simulink model "sim_autotrans"  (R2018b)
settings: Solver=ode5  StartTime=0.0  StopTime=30  RelTol=1e-3  AbsTol=1e-6
PostLoadFcn:
  | removeModelListener(bdroot(gcs))
InitFcn:
  | [listenerNodes] = setupModelListener(gcs);
StopFcn:
  | runModelCoverage(gcs,listenerNodes,dataObj,ChartObj,stateFlowCov,groupCharts,1)
model workspace (MAT data in the model file):
  CONVERTER_DATA = [0  137.465208994  2.232; 0.1  137.065019157  2.075; 0.2  135.864449646  1.975; 0.3  135.664354728  1.846; 0.4  137.565256453  1.72; 0.5  140.366585312  1.564; 0.6  145.268910814  1.409; 0.7  152.872517717  1.254; 0.8  162.9773111  1.096; 0.81  164.27792807  1.08; 0.82  166.178829795  1.061; 0.83  167.979684062  1.043; 0.84  170.080680706  1.028; 0.85  172.781962105  1.012; 0.86  175.383196045  1.002; 0.87  179.585189333  1.002; 0.88  183.587087703  1.001; 0.89  189.890077635  0.998; 0.9  197.693779455  0.999; 0.92  215.902417037  1.001; 0.94  244.515990379  1.002]
  DOWN_TABLE = [0  5  20  35; 0  5  20  35; 0  5  25  40; 0  5  30  50; 0  30  50  80; 0  30  50  80]
  DOWN_TH_BP = [0; 5; 40; 50; 90; 100]
  EMAP = [-40  -44  -49  -53  -57  -61  -65  -70  -74  -78  -82; 215  117  85  66  44  29  10  -2  -13  -22  -32; 245  208  178  148  122  104  85  66  48  33  18; 264  260  241  219  193  167  152  133  119  96  85; 264  279  282  275  260  238  223  208  189  171  152; 267  290  293  297  290  275  260  256  234  212  193; 267  297  305  305  305  301  293  282  267  249  226; 267  301  308  312  319  323  319  316  297  279  253; 267  301  312  319  327  327  327  327  312  293  267; 267  301  312  319  327  334  334  334  319  305  275]
  Iei = 0.0219914882836
  NE_VEC = [800 1200 1600 2000 2400 2800 3200 3600 4000 4400 4800]
  TH_VEC = [0; 20; 30; 40; 50; 60; 70; 80; 90; 100]
  TWAIT = 2
  UP_TABLE = [10  30  50  1000000; 10  30  50  1000000; 15  30  50  1000000; 23  41  60  1000000; 40  70  100  1000000; 40  70  100  1000000]
  UP_TH_BP = [0; 25; 35; 50; 90; 100]
  VEHICLE_DATA = [3.23; 40; 0.02; 1; 12.0941478573; 0]
undefined symbols (not defined in the file): sigbuilder_block
Description:
  | Modeling an Automatic Transmission Controller
  | 
  | In this example, Simulink(R) is used to model an automotive drivetrain. Stateflow(R)
  | enhances the Simulink model with its representation of the transmission
  | control logic. Simulink provides a powerful environment for the modeling and
  | simulation of dynamic systems and processes. In many systems, though,
  | supervisory functions like changing modes or invoking new gain schedules must
  | respond to events that may occur and conditions that develop over time. As a
  | result, the environment requires a language capable of managing these multiple
  | modes and developing conditions. In the following example, Stateflow
  | demonstrates its strength in this capacity by performing the function of gear
  | selection in an automatic transmission. This function is combined with the
  | drivetrain dynamics in a natural and intuitive manner by incorporating a
  | Stateflow block in the Simulink block diagram.
settings Model: DataTypeOverride=Double  MinMaxOverflowLogging=ForceOff  FPTRunName=Active  PauseTimes=15  ExtModeTrigMode=oneshot  ExtModeArmWhenConnect=off  ExtModeAutoUpdateStatusClock=off  Creator=The MathWorks, Inc.  LastModifiedBy=nacnm6
settings SolverCC: AutoScaleAbsTol=off
settings DataIOCC: SaveFormat=StructureWithTime  SaveOutput=off  SaveTime=off  SignalLoggingName=Harness_Signal_Log
settings OptimizationCC: BlockReduction=off  ExpressionDepthLimit=2147483647  InitFltsAndDblsToZero=on  LifeSpan=inf
settings DebuggingCC: SignalInfNanChecking=error  ReadBeforeWriteMsg=DisableAll  WriteAfterWriteMsg=DisableAll  WriteAfterReadMsg=DisableAll  SaveWithParameterizedLinksMsg=none  CheckExecutionContextPreStartOutputMsg=on  CheckExecutionContextRuntimeOutputMsg=on  MultiTaskCondExecSysMsg=none  SigSpecEnsureSampleTimeMsg=none  IntegerOverflowMsg=none  FcnCallInpInsideContextMsg=warning  SignalLabelMismatchMsg=error  UnconnectedInputMsg=error  UnconnectedOutputMsg=error  UnconnectedLineMsg=error  UniqueDataStoreMsg=error  BusObjectLabelMismatch=error  RootOutportRequireBusObject=error  AllowSymbolicDim=off  StateNameClashWarn=warning  StrictBusMsg=ErrorOnBusTreatedAsVector  NonBusSignalsTreatedAsBus=error  SFUnexpectedBacktrackingDiag=warning  SFNoUnconditionalDefaultTransitionDiag=warning  SFExecutionAtInitializationDiag=none  IntegerSaturationMsg=none
settings HardwareCC: ProdBitPerPointer=32  ProdBitPerSizeT=32  ProdBitPerPtrDiffT=32  ProdLargestAtomicFloat=None  ProdIntDivRoundTo=Floor  ProdEndianess=Unspecified  ProdWordSize=32  ProdHWDeviceType=32-bit Generic
settings ModelReferenceCC: PropagateSignalLabelsOutOfModel=off
settings SFSimCC: SFSimEcho=off  SimUseLocalCustomCode=off  SimParseCustomCode=off
settings RTWCC: RTWUseLocalCustomCode=off
settings CodeAppCC: StateflowObjectComments=on
settings GRTTargetCC: TargetFcnLib=ansi_tfl_tmw.mat  TargetLangStandard=C89/C90 (ANSI)  GeneratePreprocessorConditionals=Disable all  CombineOutputUpdateFcns=off  GRTInterface=on
settings ConfigComp: CovMetricSettings=dcmtr  CovHTMLOptions=-aTS=1 -bRG=1 -bTC=1 -hTR=0 -nFC=0 -scm=1 -bcm=1 -xEv=0  CovSaveCumulativeToWorkspaceVar=on  CovSaveSingleToWorkspaceVar=on  CovExternalEMLEnable=off

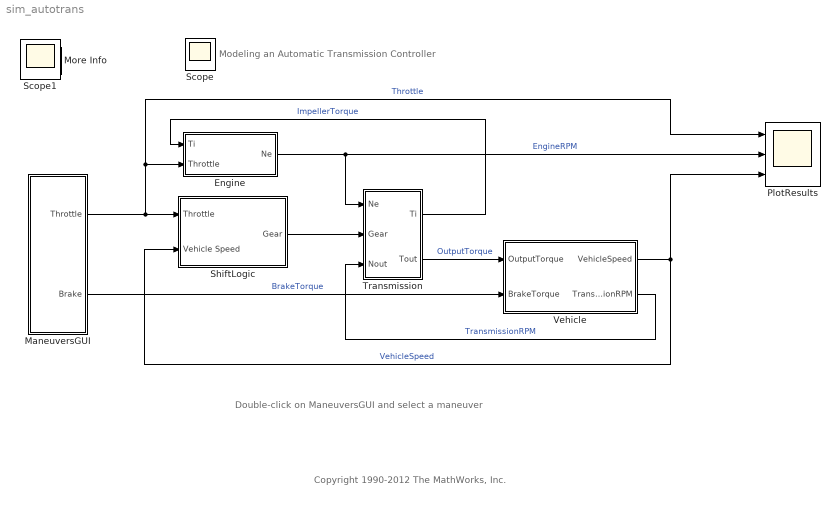
== system sim_autotrans ==
  note: Double-click on ManeuversGUI and select a maneuver
  note: Modeling an Automatic Transmission Controller
  note: Copyright 1990-2012 The MathWorks, Inc.
  Engine : Subsystem
  ManeuversGUI : Subsystem  Tag=STV Subsys  LoadFcn=sigbuilder_block('load');  StartFcn=sigbuilder_block('start');  StopFcn=sigbuilder_block('stop');  ClipboardFcn=sigbuilder_block('clipboard');  mask(Sigbuilder block){tuvar=[0:10]}
      mask help: Sigbuilder GUI
      mask init:
      | tuvar = sigbuilder_block('maskInit');
      settings: CopyFcn=sigbuilder_block('copy');  DeleteFcn=sigbuilder_block('delete');  ModelCloseFcn=sigbuilder_block('modelClose');  PreSaveFcn=sigbuilder_block('preSave');  PauseFcn=sigbuilder_block('pause')  ContinueFcn=sigbuilder_block('continue')  NameChangeFcn=sigbuilder_block('namechange');  OpenFcn=sigbuilder_block('open',[80.8 328 413.6 257.6 ]);  CloseFcn=sigbuilder_block('close');
      mask Display: plot(0, 0, 100, 100,[2, 2, 32, 32, 2], [68, 8, 8, 68, 68],[32, 2], [38, 38], [32, 19, 2],[53, 60, 44], [32, 17, 17, 2],[16, 16, 31, 31]);txt = getActiveGroup(gcbh);text(2, 100, txt,'verticalAlignment', 'top');
  More Info : Subsystem
      settings: OpenFcn=showdemo(bdroot(gcb))
      mask Display: disp('?')
  PlotResults : Scope  NumInputPorts=3
  ShiftLogic : Subsystem  TreatAsAtomicUnit=on  SystemSampleTime=0.04
  Transmission : Subsystem
  Vehicle : Subsystem  mask(vehicle model){Rfd=VEHICLE_DATA(1), rload0=VEHICLE_DATA(2), rload2=VEHICLE_DATA(3), Rw=VEHICLE_DATA(4), Iv=VEHICLE_DATA(5), N20=VEHICLE_DATA(6)/VEHICLE_DATA(4)*VEHICLE_DATA(1)}
      mask prompts: Rfd "final drive ratio"; rload0 "drag friction at wheels"; rload2 "aerodynamic drag"; Rw "wheel radius"; Iv "vehicle inertia"; N20 "initial transmission output speed"
      mask help: vehicle dynamics: torque input from trans., outputs are input speed (transmission output) and vehicle speed
      mask Display: image([matlabroot,'/toolbox/simulink/simdemos/automotive/html/NSX_3Colors.jpg'])
  Scope : Scope
  Scope1 : Scope
  wires:
  Transmission/1(Ti) -> Engine/1(Ti)  "ImpellerTorque"
  Engine/1(Ne) -> Transmission/1(Ne), PlotResults/2  "EngineRPM"
  Transmission/2(Tout) -> Vehicle/1(OutputTorque)  "OutputTorque"
  Vehicle/2(TransmissionRPM) -> Transmission/3(Nout)  "TransmissionRPM"
  ShiftLogic/1(Gear) -> Transmission/2(Gear)
  Vehicle/1(VehicleSpeed) -> PlotResults/3, ShiftLogic/2(Vehicle Speed)  "VehicleSpeed"
  ManeuversGUI/1(Throttle) -> ShiftLogic/1(Throttle), Engine/2(Throttle), PlotResults/1  "Throttle"
  ManeuversGUI/2(Brake) -> Vehicle/2(BrakeTorque)  "BrakeTorque"

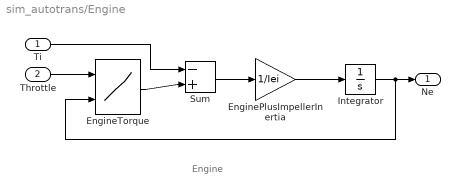
== system sim_autotrans/Engine ==
  note: Engine
  Ti : Inport
  Throttle : Inport  Port=2
  EnginePlusImpellerInertia : Gain  Gain=1/Iei  SaturateOnIntegerOverflow=on  OutDataTypeStr=Inherit: Same as input  ParamDataTypeStr=Inherit: Same as input
  EngineTorque : Lookup_n-D  BreakpointsForDimension1=TH_VEC  BreakpointsForDimension2=NE_VEC  Table=EMAP  InputSameDT=on
  Integrator : Integrator  InitialCondition=1000  LimitOutput=on  UpperSaturationLimit=6000  LowerSaturationLimit=600  ZeroCross=off
  Sum : Sum  Inputs=-+  SaturateOnIntegerOverflow=on  InputSameDT=on  OutDataTypeStr=Inherit: Same as first input
  Ne : Outport
  wires:
  Ti/1 -> Sum/1
  Throttle/1 -> EngineTorque/1
  Integrator/1 -> EngineTorque/2, Ne/1
  Sum/1 -> EnginePlusImpellerInertia/1
  EnginePlusImpellerInertia/1 -> Integrator/1
  EngineTorque/1 -> Sum/2

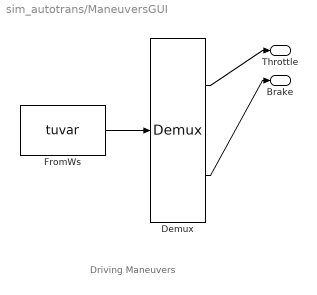
== system sim_autotrans/ManeuversGUI ==
  note: Driving Maneuvers
  Demux : Demux  Tag=STV Demux  Outputs=2
  FromWs : FromWorkspace  Tag=STV FromWs  VariableName=tuvar  SampleTime=0
      SigBuilderData=|
      | dataSet(1).timeRange = [0 50]
      | dataSet(1).name = 'Passing Maneuver'
      | dataSet(2).timeRange = [0 50]
      | dataSet(2).name = 'Gradual Acceleration'
      | dataSet(3).timeRange = [0 50]
      | dataSet(3).name = 'Hard braking'
      | dataSet(4).timeRange = [0 50]
      | dataSet(4).name = 'Coasting'
      | sbobj.Groups(1).Name = 'Passing Maneuver'
      | sbobj.Groups(1).Signals(1).Name = 'Throttle'
      | sbobj.Groups(1).Signals(1).XData = [0 14.9 15 50]
      | sbobj.Groups(1).Signals(1).YData = [60 40 100 58.8235294118]
      | sbobj.Groups(1).Signals(2).Name = 'Brake'
      | sbobj.Groups(1).Signals(2).XData = [0 50]
      | sbobj.Groups(1).Signals(2).YData = [0 0]
      | sbobj.Groups(2).Name = 'Gradual Acceleration'
      | sbobj.Groups(2).Signals(1).Name = 'Throttle'
      | sbobj.Groups(2).Signals(1).XData = [0 50]
      | sbobj.Groups(2).Signals(1).YData = [13.4 24]
      | sbobj.Groups(2).Signals(2).Name = 'Brake'
      | sbobj.Groups(2).Signals(2).XData = [0 50]
      | sbobj.Groups(2).Signals(2).YData = [0 0]
      | sbobj.Groups(3).Name = 'Hard braking'
      | sbobj.Groups(3).Signals(1).Name = 'Throttle'
      | sbobj.Groups(3).Signals(1).XData = [0 5.1 5.1 50]
      | sbobj.Groups(3).Signals(1).YData = [50 50 1 1]
      | sbobj.Groups(3).Signals(2).Name = 'Brake'
      | sbobj.Groups(3).Signals(2).XData = [0 10 10 50]
      | sbobj.Groups(3).Signals(2).YData = [0 0 325 325]
      | sbobj.Groups(4).Name = 'Coasting'
      | sbobj.Groups(4).Signals(1).Name = 'Throttle'
      | sbobj.Groups(4).Signals(1).XData = [0 4.8 4.8 50]
      | sbobj.Groups(4).Signals(1).YData = [80 80 1 1]
      | sbobj.Groups(4).Signals(2).Name = 'Brake'
      | sbobj.Groups(4).Signals(2).XData = [0 50]
      | sbobj.Groups(4).Signals(2).YData = [0 0]
  Throttle : Outport  Tag=STV Outport
  Brake : Outport  Tag=STV Outport  Port=2
  wires:
  FromWs/1 -> Demux/1
  Demux/1 -> Throttle/1
  Demux/2 -> Brake/1

== system sim_autotrans/More Info ==

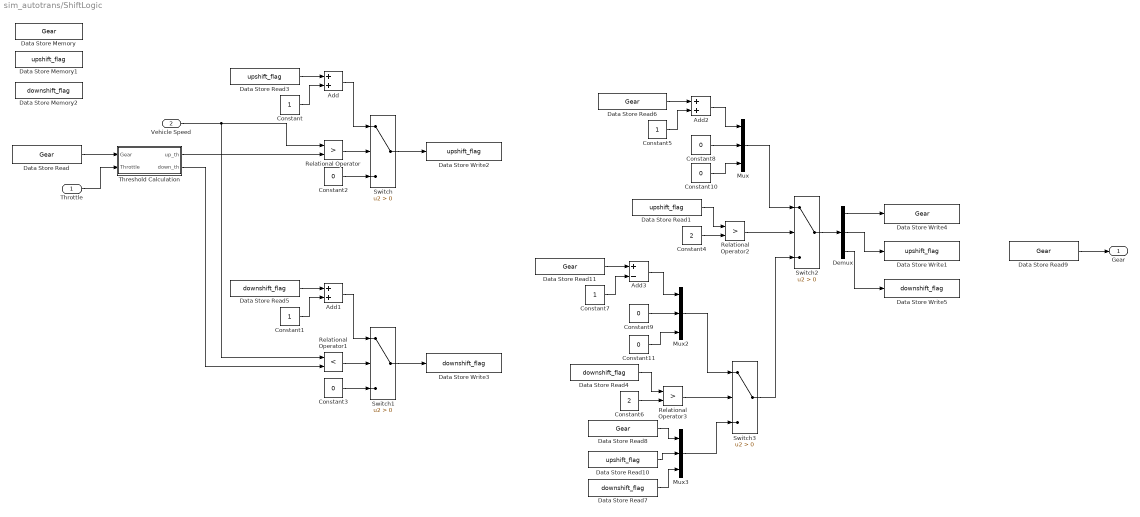
== system sim_autotrans/ShiftLogic ==
  Throttle : Inport
  Vehicle Speed : Inport  Port=2
  Add : Sum
  Add1 : Sum
  Add2 : Sum
  Add3 : Sum  Inputs=+-
  Constant{,1,5,7} (4 alike) : Constant
  Constant{2..3,8..11} (6 alike) : Constant  Value=0
  Constant4 : Constant  Value=2
  Constant6 : Constant  Value=2
  Data Store Memory : DataStoreMemory  Priority=1  DataStoreName=Gear  ReadBeforeWriteMsg=warning  WriteAfterWriteMsg=warning  WriteAfterReadMsg=warning  InitialValue=1  ShowAdditionalParam=off
      settings: AttributesFormatString=Priority: %<Priority>
  Data Store Memory1 : DataStoreMemory  Priority=1  DataStoreName=upshift_flag  ReadBeforeWriteMsg=warning  WriteAfterWriteMsg=warning  WriteAfterReadMsg=warning  ShowAdditionalParam=off
      settings: AttributesFormatString=Priority: %<Priority>
  Data Store Memory2 : DataStoreMemory  Priority=1  DataStoreName=downshift_flag  ReadBeforeWriteMsg=warning  WriteAfterWriteMsg=warning  WriteAfterReadMsg=warning  ShowAdditionalParam=off
      settings: AttributesFormatString=Priority: %<Priority>
  Data Store Read{,6,8,11} (4 alike) : DataStoreRead  Priority=10  DataStoreName=Gear
      settings: AttributesFormatString=Priority: %<Priority>
  Data Store Read1 : DataStoreRead  Priority=30  DataStoreName=upshift_flag
      settings: AttributesFormatString=Priority: %<Priority>
  Data Store Read10 : DataStoreRead  Priority=30  DataStoreName=upshift_flag
      settings: AttributesFormatString=Priority: %<Priority>
  Data Store Read3 : DataStoreRead  Priority=10  DataStoreName=upshift_flag
      settings: AttributesFormatString=Priority: %<Priority>
  Data Store Read4 : DataStoreRead  Priority=30  DataStoreName=downshift_flag
      settings: AttributesFormatString=Priority: %<Priority>
  Data Store Read5 : DataStoreRead  Priority=10  DataStoreName=downshift_flag
      settings: AttributesFormatString=Priority: %<Priority>
  Data Store Read7 : DataStoreRead  Priority=30  DataStoreName=downshift_flag
      settings: AttributesFormatString=Priority: %<Priority>
  Data Store Read9 : DataStoreRead  Priority=50  DataStoreName=Gear
      settings: AttributesFormatString=Priority: %<Priority>
  Data Store Write1 : DataStoreWrite  DataStoreName=upshift_flag
  Data Store Write2 : DataStoreWrite  Priority=20  DataStoreName=upshift_flag
      settings: AttributesFormatString=Priority: %<Priority>
  Data Store Write3 : DataStoreWrite  Priority=20  DataStoreName=downshift_flag
      settings: AttributesFormatString=Priority: %<Priority>
  Data Store Write4 : DataStoreWrite  Priority=40  DataStoreName=Gear
      settings: AttributesFormatString=Priority: %<Priority>
  Data Store Write5 : DataStoreWrite  DataStoreName=downshift_flag
  Demux : Demux  Outputs=3
  Mux : Mux  Inputs=3
  Mux2 : Mux  Inputs=3
  Mux3 : Mux  Inputs=3
  Relational Operator : RelationalOperator  StartFcn=|  Operator=>  OutDataTypeStr=boolean  RndMeth=Nearest
      | relationOpBlks(1) = add_exec_event_listener(gcb,'PostOutputs', @checkRuntimeData); 
      | relationOpBlks(1) = add_exec_event_listener(gcb,'PostOutputs', @checkRuntimeData); 
      | relationOpBlks(1) = add_exec_event_listener(gcb,'PostOutputs', @checkRuntimeData); 
      | relationOpBlks(1) = add_exec_event_listener(gcb,'PostOutputs', @checkRuntimeData);
  Relational Operator1 : RelationalOperator  StartFcn=|  Operator=<  OutDataTypeStr=boolean  RndMeth=Nearest
      | relationOpBlks(2) = add_exec_event_listener(gcb,'PostOutputs', @checkRuntimeData); 
      | relationOpBlks(2) = add_exec_event_listener(gcb,'PostOutputs', @checkRuntimeData); 
      | relationOpBlks(2) = add_exec_event_listener(gcb,'PostOutputs', @checkRuntimeData); 
      | relationOpBlks(2) = add_exec_event_listener(gcb,'PostOutputs', @checkRuntimeData);
  Relational Operator2 : RelationalOperator  StartFcn=|  Operator=>  OutDataTypeStr=boolean  RndMeth=Nearest
      | relationOpBlks(3) = add_exec_event_listener(gcb,'PostOutputs', @checkRuntimeData); 
      | relationOpBlks(3) = add_exec_event_listener(gcb,'PostOutputs', @checkRuntimeData); 
      | relationOpBlks(3) = add_exec_event_listener(gcb,'PostOutputs', @checkRuntimeData); 
      | relationOpBlks(3) = add_exec_event_listener(gcb,'PostOutputs', @checkRuntimeData);
  Relational Operator3 : RelationalOperator  StartFcn=|  Operator=>  OutDataTypeStr=boolean  RndMeth=Nearest
      | relationOpBlks(4) = add_exec_event_listener(gcb,'PostOutputs', @checkRuntimeData); 
      | relationOpBlks(4) = add_exec_event_listener(gcb,'PostOutputs', @checkRuntimeData); 
      | relationOpBlks(4) = add_exec_event_listener(gcb,'PostOutputs', @checkRuntimeData); 
      | relationOpBlks(4) = add_exec_event_listener(gcb,'PostOutputs', @checkRuntimeData);
  Switch : Switch  StartFcn=switchBlks(2) = add_exec_event_listener(gcb,'PostOutputs', @getRunTimeData);  Criteria=u2 > Threshold
  Switch1 : Switch  StartFcn=switchBlks(2) = add_exec_event_listener(gcb,'PostOutputs', @getRunTimeData);  Criteria=u2 > Threshold
  Switch2 : Switch  StartFcn=|  Criteria=u2 > Threshold
      | switchBlks(3) = add_exec_event_listener(gcb,'PostOutputs', @checkRuntimeData); 
      | switchBlks(3) = add_exec_event_listener(gcb,'PostOutputs', @checkRuntimeData); 
      | switchBlks(3) = add_exec_event_listener(gcb,'PostOutputs', @checkRuntimeData); 
      | switchBlks(3) = add_exec_event_listener(gcb,'PostOutputs', @checkRuntimeData);
  Switch3 : Switch  StartFcn=|  Criteria=u2 > Threshold
      | switchBlks(4) = add_exec_event_listener(gcb,'PostOutputs', @checkRuntimeData); 
      | switchBlks(4) = add_exec_event_listener(gcb,'PostOutputs', @checkRuntimeData); 
      | switchBlks(4) = add_exec_event_listener(gcb,'PostOutputs', @checkRuntimeData); 
      | switchBlks(4) = add_exec_event_listener(gcb,'PostOutputs', @checkRuntimeData);
  Threshold Calculation : Subsystem
  Gear : Outport
  wires:
  Throttle/1 -> Threshold Calculation/2(Throttle)
  Data Store Read/1 -> Threshold Calculation/1(Gear)
  Threshold Calculation/1(up_th) -> Relational Operator/2
  Relational Operator/1 -> Switch/2
  Constant/1 -> Add/2
  Add/1 -> Switch/1
  Data Store Read3/1 -> Add/1
  Vehicle Speed/1 -> Relational Operator/1, Relational Operator1/1
  Threshold Calculation/2(down_th) -> Relational Operator1/2
  Relational Operator1/1 -> Switch1/2
  Constant1/1 -> Add1/2
  Add1/1 -> Switch1/1
  Data Store Read5/1 -> Add1/1
  Constant2/1 -> Switch/3
  Constant3/1 -> Switch1/3
  Relational Operator2/1 -> Switch2/2
  Constant4/1 -> Relational Operator2/2
  Switch/1 -> Data Store Write2/1
  Switch1/1 -> Data Store Write3/1
  Data Store Read1/1 -> Relational Operator2/1
  Constant5/1 -> Add2/2
  Data Store Read6/1 -> Add2/1
  Data Store Read9/1 -> Gear/1
  Add2/1 -> Mux/1
  Mux/1 -> Switch2/1
  Switch2/1 -> Demux/1
  Demux/1 -> Data Store Write4/1
  Demux/2 -> Data Store Write1/1
  Relational Operator3/1 -> Switch3/2
  Constant6/1 -> Relational Operator3/2
  Data Store Read4/1 -> Relational Operator3/1
  Constant7/1 -> Add3/2
  Data Store Read11/1 -> Add3/1
  Add3/1 -> Mux2/1
  Mux2/1 -> Switch3/1
  Data Store Read8/1 -> Mux3/1
  Mux3/1 -> Switch3/3
  Constant8/1 -> Mux/2
  Constant9/1 -> Mux2/2
  Data Store Read7/1 -> Mux3/3
  Data Store Read10/1 -> Mux3/2
  Switch3/1 -> Switch2/3
  Demux/3 -> Data Store Write5/1
  Constant10/1 -> Mux/3
  Constant11/1 -> Mux2/3

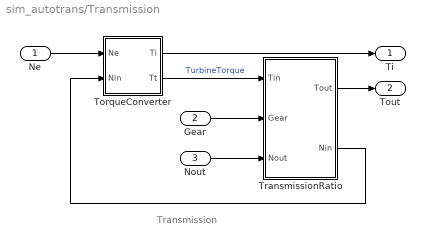
== system sim_autotrans/Transmission ==
  note: Transmission
  Ne : Inport
  Gear : Inport  Port=2
  Nout : Inport  Port=3
  TorqueConverter : Subsystem  mask(torque converter){speedratio=CONVERTER_DATA(:,1), Kfactor=CONVERTER_DATA(:,2), Torkratio=CONVERTER_DATA(:,3)}
      mask prompts: speedratio "speed ratio"; Kfactor "K factor"; Torkratio "torque ratio"
      mask help: torque converter
      mask Help: Torque converter input and output torques are computed as a function of the input and output speeds
      mask Display: plot([cos([90:10:450]*pi/180),.63*cos([90:10:450]*pi/180),.63*cos([90:10:240]*pi/180),cos([240:10:300]*pi/180),.63*cos([300]*pi/180)],[sin([90:10:450]*pi/180),.63*sin([90:10:450]*pi/180)+.1,.63*sin([90:10:240]*pi/180)+.1,sin([240:10:300]*pi/180),.63*sin([300]*pi/180)+.1])
  TransmissionRatio : Subsystem
  Ti : Outport
  Tout : Outport  Port=2
  wires:
  TransmissionRatio/1(Tout) -> Tout/1
  TorqueConverter/1(Ti) -> Ti/1
  Nout/1 -> TransmissionRatio/3(Nout)
  Gear/1 -> TransmissionRatio/2(Gear)
  Ne/1 -> TorqueConverter/1(Ne)
  TransmissionRatio/2(Nin) -> TorqueConverter/2(Nin)
  TorqueConverter/2(Tt) -> TransmissionRatio/1(Tin)  "TurbineTorque"

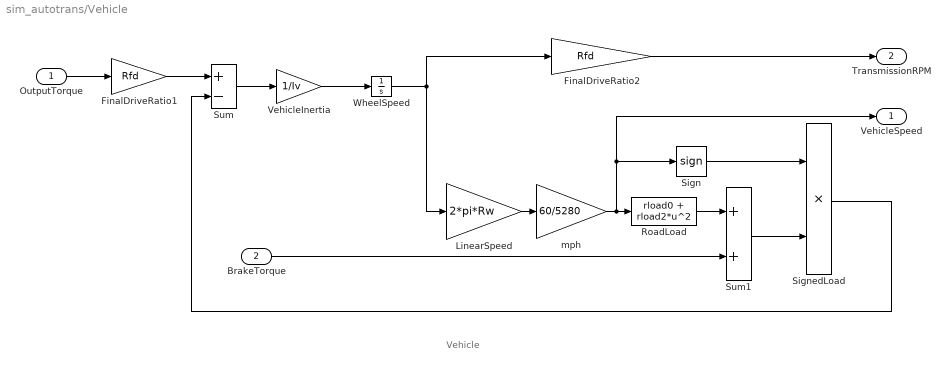
== system sim_autotrans/Vehicle ==
  note: Vehicle
  OutputTorque : Inport
  BrakeTorque : Inport  Port=2
  FinalDriveRatio1 : Gain  Gain=Rfd  SaturateOnIntegerOverflow=on  OutDataTypeStr=Inherit: Same as input  ParamDataTypeStr=Inherit: Same as input
  FinalDriveRatio2 : Gain  Gain=Rfd  SaturateOnIntegerOverflow=on  OutDataTypeStr=Inherit: Same as input  ParamDataTypeStr=Inherit: Same as input
  LinearSpeed : Gain  Gain=2*pi*Rw  SaturateOnIntegerOverflow=on  OutDataTypeStr=Inherit: Same as input  ParamDataTypeStr=Inherit: Same as input
  RoadLoad : Fcn  Expr=rload0 + rload2*u^2
  Sign : Signum
  SignedLoad : Product  SaturateOnIntegerOverflow=on  InputSameDT=on  OutDataTypeStr=Inherit: Same as first input
  Sum : Sum  Inputs=+-  SaturateOnIntegerOverflow=on  InputSameDT=on  OutDataTypeStr=Inherit: Same as first input
  Sum1 : Sum  SaturateOnIntegerOverflow=on  InputSameDT=on  OutDataTypeStr=Inherit: Same as first input
  VehicleInertia : Gain  Gain=1/Iv  SaturateOnIntegerOverflow=on  OutDataTypeStr=Inherit: Same as input  ParamDataTypeStr=Inherit: Same as input
  WheelSpeed : Integrator  InitialCondition=N20/Rfd  ZeroCross=off
  mph : Gain  Gain=60/5280  SaturateOnIntegerOverflow=on  OutDataTypeStr=Inherit: Same as input  ParamDataTypeStr=Inherit: Same as input
  VehicleSpeed : Outport
  TransmissionRPM : Outport  Port=2
  wires:
  FinalDriveRatio2/1 -> TransmissionRPM/1
  BrakeTorque/1 -> Sum1/2
  Sum1/1 -> SignedLoad/2
  RoadLoad/1 -> Sum1/1
  Sign/1 -> SignedLoad/1
  SignedLoad/1 -> Sum/2
  OutputTorque/1 -> FinalDriveRatio1/1
  VehicleInertia/1 -> WheelSpeed/1
  Sum/1 -> VehicleInertia/1
  mph/1 -> VehicleSpeed/1, Sign/1, RoadLoad/1
  LinearSpeed/1 -> mph/1
  WheelSpeed/1 -> LinearSpeed/1, FinalDriveRatio2/1
  FinalDriveRatio1/1 -> Sum/1

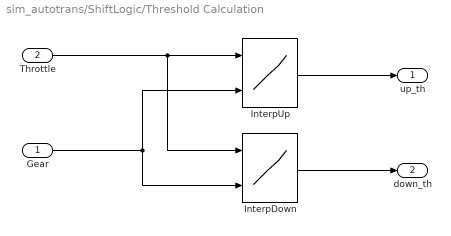
== system sim_autotrans/ShiftLogic/Threshold Calculation ==
  Gear : Inport
  Throttle : Inport  Port=2
  InterpDown : Lookup_n-D  BreakpointsForDimension1=DOWN_TH_BP  BreakpointsForDimension2=[1:4]  Table=DOWN_TABLE  OutDataTypeStr=double  LockScale=on
  InterpUp : Lookup_n-D  BreakpointsForDimension1=UP_TH_BP  BreakpointsForDimension2=[1:4]  Table=UP_TABLE  OutDataTypeStr=double  LockScale=on
  up_th : Outport  InitialOutput=0
  down_th : Outport  Port=2  InitialOutput=0
  wires:
  Gear/1 -> InterpUp/2, InterpDown/2
  Throttle/1 -> InterpUp/1, InterpDown/1
  InterpDown/1 -> down_th/1
  InterpUp/1 -> up_th/1

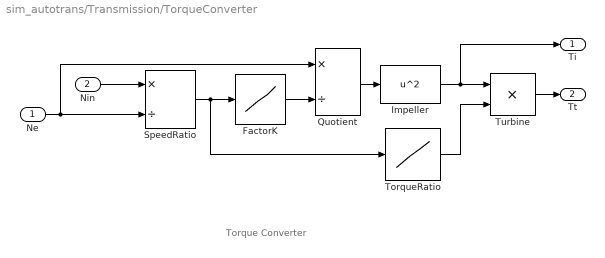
== system sim_autotrans/Transmission/TorqueConverter ==
  note: Torque Converter
  Ne : Inport
  Nin : Inport  Port=2
  FactorK : Lookup_n-D  NumberOfTableDimensions=1  BreakpointsForDimension1=speedratio  Table=Kfactor  SaturateOnIntegerOverflow=on  InputSameDT=on
  Impeller : Fcn  Expr=u^2
  Quotient : Product  Inputs=*/  SaturateOnIntegerOverflow=on  InputSameDT=on  OutDataTypeStr=Inherit: Same as first input
  SpeedRatio : Product  Inputs=*/  SaturateOnIntegerOverflow=on  InputSameDT=on  OutDataTypeStr=Inherit: Same as first input
  TorqueRatio : Lookup_n-D  NumberOfTableDimensions=1  BreakpointsForDimension1=speedratio  Table=Torkratio  SaturateOnIntegerOverflow=on  InputSameDT=on
  Turbine : Product  SaturateOnIntegerOverflow=on  InputSameDT=on  OutDataTypeStr=Inherit: Same as first input
  Ti : Outport
  Tt : Outport  Port=2
  wires:
  TorqueRatio/1 -> Turbine/2
  Quotient/1 -> Impeller/1
  FactorK/1 -> Quotient/2
  SpeedRatio/1 -> TorqueRatio/1, FactorK/1
  Impeller/1 -> Turbine/1, Ti/1
  Turbine/1 -> Tt/1
  Ne/1 -> SpeedRatio/2, Quotient/1
  Nin/1 -> SpeedRatio/1

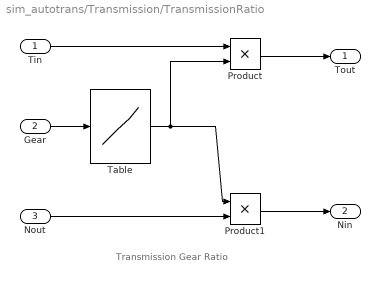
== system sim_autotrans/Transmission/TransmissionRatio ==
  note: Transmission Gear Ratio
  Tin : Inport
  Gear : Inport  Port=2
  Nout : Inport  Port=3
  Product : Product  SaturateOnIntegerOverflow=on  InputSameDT=on  OutDataTypeStr=Inherit: Same as first input
  Product1 : Product  SaturateOnIntegerOverflow=on  InputSameDT=on  OutDataTypeStr=Inherit: Same as first input
  Table : Lookup_n-D  NumberOfTableDimensions=1  BreakpointsForDimension1=[1 2 3 4]  Table=[2.393 1.450 1.000 0.677]  OutDataTypeStr=double  SaturateOnIntegerOverflow=on  InputSameDT=on  LockScale=on
  Tout : Outport
  Nin : Outport  Port=2
  wires:
  Table/1 -> Product1/1, Product/2
  Nout/1 -> Product1/2
  Product1/1 -> Nin/1
  Product/1 -> Tout/1
  Tin/1 -> Product/1
  Gear/1 -> Table/1
